simulink model "prystupalab5_si"  (R2023b)
settings: Solver=VariableStepAuto  StartTime=0.0  StopTime=10.0  MaxStep=0.01  RelTol=1e-3
values from neighbouring files (symbols this model uses):
  a = 1    [prystupalab5.m]    (also in prystupalab5_1.m)
  b = omega(1)^2    [prystupalab5.m]    (also in prystupalab5_1.m = omega(i)^2)
  du = 1    [prystupalab5.m]    (also in prystupalab5_1.m)
  ksi = tabelaksi(i)    [prystupalab5.m]    (also in prystupalab5_1.m)
  t0 = 0    [prystupalab5.m]    (also in prystupalab5_1.m)
  ts = 10    [prystupalab5.m]    (also in prystupalab5_1.m)
  u0 = 0    [prystupalab5.m]    (also in prystupalab5_1.m)
  w = omega(1)    [prystupalab5.m]    (also in prystupalab5_1.m = omega1(i))
settings Model: Creator=Adam  LastModifiedBy=Adam

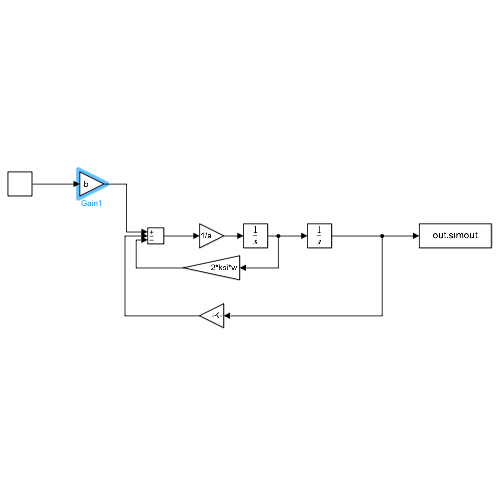
[thumbnail: Simulink's stored preview of the top-level diagram]
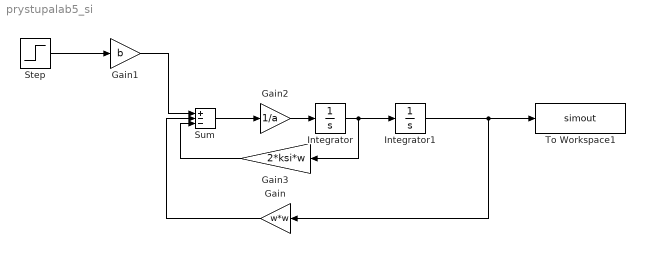
== system prystupalab5_si ==
  Gain : Gain  Gain=w*w
  Gain1 : Gain  Gain=b
  Gain2 : Gain  Gain=1/a
  Gain3 : Gain  Gain=2*ksi*w
  Integrator : Integrator
  Integrator1 : Integrator
  Step : Step  Time=t0  Before=u0  After=u0+du  SampleTime=ts
  Sum : Sum  Inputs=+--
  To Workspace1 : ToWorkspace  VariableName=simout  SampleTime=-1
  wires:
  Gain3/1 -> Sum/3
  Step/1 -> Gain1/1
  Integrator/1 -> Gain3/1, Integrator1/1
  Gain1/1 -> Sum/1
  Gain/1 -> Sum/2
  Gain2/1 -> Integrator/1
  Integrator1/1 -> To Workspace1/1, Gain/1
  Sum/1 -> Gain2/1
